simulink model "controladorLQR"  (Simulink 7.9)
settings: Solver=ode45  StartTime=0.0  StopTime=10  MaxStep=0.03  MinStep=0.01  RelTol=1e-3
values from neighbouring files (symbols this model uses):
  InicialCondition = [x0;theta0*pi/180;xvel0;thetaVel0]    [loadModelParameters.m]
  K = lqr(A,B,Q,R)    [LQR.m]    (also in bestQ.m = setK_lqr(Q_i); graficosPenduloReal.m = setK_lqr(Q_optimo))
settings Model: Creator=Daniel  LastModifiedBy=root
settings SolverCC: InitialStep=0.01
settings DebuggingCC: FcnCallInpInsideContextMsg=Use local settings  StrictBusMsg=Warning
settings SFSimCC: SimParseCustomCode=off
settings GRTTargetCC: CombineOutputUpdateFcns=off  GRTInterface=on

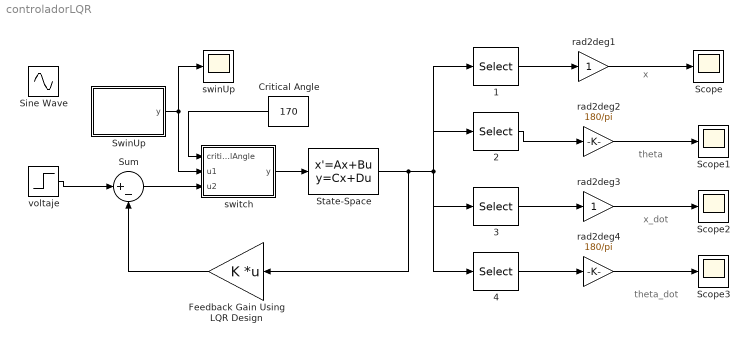
== system controladorLQR ==
  note: x
  note: theta
  note: theta_dot
  note: x_dot
  " 1" : Selector  InputPortWidth=4  IndexOptions=Index vector (dialog)  Indices=1  OutputSizes=1
  " 2" : Selector  InputPortWidth=4  IndexOptions=Index vector (dialog)  Indices=2  OutputSizes=1
  " 3" : Selector  InputPortWidth=4  IndexOptions=Index vector (dialog)  Indices=3  OutputSizes=1
  " 4" : Selector  InputPortWidth=4  IndexOptions=Index vector (dialog)  Indices=4  OutputSizes=1
  Critical Angle : Constant  Value=170
  Feedback Gain Using LQR Design : Gain  Gain=K  Multiplication=Matrix(K*u) (u vector)
  Scope{,1..3} (4 alike) : Scope
      Scope2 settings: SaveName=ScopeData2
      Scope3 settings: SaveName=ScopeData3
  Sine Wave : Sin  SampleTime=0
  State-Space : StateSpace  A="[0 0 1 0; 0 0 0 1; 0 0.5401 -0.7235 0; 0  14.955 -0.9854 0]"  B="[0  ;0 ;2.2747 ;3.0978]"  C=eye(4)  D=[0;0;0;0]  X0=InicialCondition
  Sum : Sum  Inputs=|+-
  SwinUp : MATLAB Function  TreatAsAtomicUnit=on
  rad2deg1 : Gain  SaturateOnIntegerOverflow=on  OutDataTypeStr=Inherit: Same as input  ParamDataTypeStr=Inherit: Same as input
  rad2deg2 : Gain  Gain=180/pi  SaturateOnIntegerOverflow=on  OutDataTypeStr=Inherit: Same as input  ParamDataTypeStr=Inherit: Same as input
  rad2deg3 : Gain  SaturateOnIntegerOverflow=on  OutDataTypeStr=Inherit: Same as input  ParamDataTypeStr=Inherit: Same as input
  rad2deg4 : Gain  Gain=180/pi  SaturateOnIntegerOverflow=on  OutDataTypeStr=Inherit: Same as input  ParamDataTypeStr=Inherit: Same as input
  swinUp : Scope
      settings: SaveName=ScopeData4
  switch : MATLAB Function  TreatAsAtomicUnit=on
  voltaje : Step  Time=0  After=0  SampleTime=0
  wires:
  " 1"/1 -> rad2deg1/1
  " 2"/1 -> rad2deg2/1
  rad2deg4/1 -> Scope3/1
  rad2deg2/1 -> Scope1/1
  rad2deg1/1 -> Scope/1
  State-Space/1 -> " 1"/1, " 3"/1, " 2"/1, " 4"/1, Feedback Gain Using LQR Design/1
  " 4"/1 -> rad2deg4/1
  switch/1(y) -> State-Space/1
  voltaje/1 -> Sum/1
  SwinUp/1(y) -> switch/2(u1), swinUp/1
  Critical Angle/1 -> switch/1(criticalAngle)
  Sum/1 -> switch/3(u2)
  " 3"/1 -> rad2deg3/1
  rad2deg3/1 -> Scope2/1
  Feedback Gain Using LQR Design/1 -> Sum/2

== matlab function switch ==
  data: criticalAngle input double; u1 input double; y output double; u2 input double
function y = fcn(criticalAngle, u1,u2)
%#eml
if (abs(u2) < criticalAngle)
    y = u2;
else
    y = u2;
end

== matlab function SwinUp ==
  data: y output double
function y = fcn()
%Funcion periodica de exitación
Ts=0.1;             % Periodo señal [s]
f=1/Ts;             % Frecuencia señal [Hz]
A = 2;               % Amplirud [V]

dt=Ts/10;           % 'Tiempo de muestreo'. Debe ser menor que el periodo de la señal
t=0:dt:30*Ts;       % Base de tiempo para la señal [s]. (se veran 30 ciclos)

u=A*sin(2*pi*f*t);  % Señal portadora con base de tiempo para visualizar la forma de la señal

y = u;
end
